simulink model "SimpleEKF_2007a"  (Simulink 6.6)
settings: Solver=FixedStepDiscrete  StartTime=0.0  StopTime=300  FixedStep=0.01  RelTol=1e-3
values from neighbouring files (symbols this model uses):
  initP = diag([ 1 1 1 1e5 1e5 1 1e5 1e5 1e5 ])    [SimpleEKF_init.m.m]
undefined symbols (not defined in the file or in its folder): DiscIntNeverNeededParam, gcbh, hwbcalib_subsystem
libraries: simulink x8, dspmtrx3 x5, dspinverses x1
(part 9 of 9)

== system SimpleEKF_2007a/INS/Attitude update/Stage2/Subsystem/a21/product1 ==
  1 : Inport  OutDataType=fixdt(1,16,0)  OutScaling=[]
  2 : Inport  Port=2  OutDataType=fixdt(1,16,0)  OutScaling=[]
  Product_1 : Product  OutDataType=fixdt(1,16,0)  OutScaling=[]  RndMeth=Zero  InputSameDT=on
  1000 : Outport  OutDataType=fixdt(1,16,0)  OutScaling=[]
  wires:
  Product_1/1 -> 1000/1
  1/1 -> Product_1/1
  2/1 -> Product_1/2

== system SimpleEKF_2007a/INS/Attitude update/Stage2/Subsystem/a21/sum ==
  1 : Inport  OutDataType=fixdt(1,16,0)  OutScaling=[]
  2 : Inport  Port=2  OutDataType=fixdt(1,16,0)  OutScaling=[]
  Sum_1 : Sum  Inputs=-+  OutDataType=fixdt(1,16,0)  OutScaling=[]  RndMeth=Zero  InputSameDT=on
  1000 : Outport  OutDataType=fixdt(1,16,0)  OutScaling=[]
  wires:
  Sum_1/1 -> 1000/1
  1/1 -> Sum_1/1
  2/1 -> Sum_1/2

== system SimpleEKF_2007a/INS/Attitude update/Stage2/Subsystem/a22/BorderBottom ==

== system SimpleEKF_2007a/INS/Attitude update/Stage2/Subsystem/a22/BorderLeft ==

== system SimpleEKF_2007a/INS/Attitude update/Stage2/Subsystem/a22/BorderRight ==

== system SimpleEKF_2007a/INS/Attitude update/Stage2/Subsystem/a22/BorderTop ==

== system SimpleEKF_2007a/INS/Attitude update/Stage2/Subsystem/a22/Subsystem Revision ==

== system SimpleEKF_2007a/INS/Attitude update/Stage2/Subsystem/a22/deMux ==
  Dmx : Inport  OutDataType=fixdt(1,16,0)  OutScaling=[]
  999 : Demux
  1 : Outport  OutDataType=fixdt(1,16,0)  OutScaling=[]
  2 : Outport  Port=2  OutDataType=fixdt(1,16,0)  OutScaling=[]
  3 : Outport  Port=3  OutDataType=fixdt(1,16,0)  OutScaling=[]
  4 : Outport  Port=4  OutDataType=fixdt(1,16,0)  OutScaling=[]
  wires:
  999/1 -> 1/1
  999/2 -> 2/1
  Dmx/1 -> 999/1
  999/3 -> 3/1
  999/4 -> 4/1

== system SimpleEKF_2007a/INS/Attitude update/Stage2/Subsystem/a22/product ==
  1 : Inport  OutDataType=fixdt(1,16,0)  OutScaling=[]
  2 : Inport  Port=2  OutDataType=fixdt(1,16,0)  OutScaling=[]
  Product_1 : Product  OutDataType=fixdt(1,16,0)  OutScaling=[]  RndMeth=Zero  InputSameDT=on
  1000 : Outport  OutDataType=fixdt(1,16,0)  OutScaling=[]
  wires:
  Product_1/1 -> 1000/1
  1/1 -> Product_1/1
  2/1 -> Product_1/2

== system SimpleEKF_2007a/INS/Attitude update/Stage2/Subsystem/a22/product1 ==
  1 : Inport  OutDataType=fixdt(1,16,0)  OutScaling=[]
  2 : Inport  Port=2  OutDataType=fixdt(1,16,0)  OutScaling=[]
  Product_1 : Product  OutDataType=fixdt(1,16,0)  OutScaling=[]  RndMeth=Zero  InputSameDT=on
  1000 : Outport  OutDataType=fixdt(1,16,0)  OutScaling=[]
  wires:
  Product_1/1 -> 1000/1
  1/1 -> Product_1/1
  2/1 -> Product_1/2

== system SimpleEKF_2007a/INS/Attitude update/Stage2/Subsystem/a22/product2 ==
  1 : Inport  OutDataType=fixdt(1,16,0)  OutScaling=[]
  2 : Inport  Port=2  OutDataType=fixdt(1,16,0)  OutScaling=[]
  Product_1 : Product  OutDataType=fixdt(1,16,0)  OutScaling=[]  RndMeth=Zero  InputSameDT=on
  1000 : Outport  OutDataType=fixdt(1,16,0)  OutScaling=[]
  wires:
  Product_1/1 -> 1000/1
  1/1 -> Product_1/1
  2/1 -> Product_1/2

== system SimpleEKF_2007a/INS/Attitude update/Stage2/Subsystem/a22/product3 ==
  1 : Inport  OutDataType=fixdt(1,16,0)  OutScaling=[]
  2 : Inport  Port=2  OutDataType=fixdt(1,16,0)  OutScaling=[]
  Product_1 : Product  OutDataType=fixdt(1,16,0)  OutScaling=[]  RndMeth=Zero  InputSameDT=on
  1000 : Outport  OutDataType=fixdt(1,16,0)  OutScaling=[]
  wires:
  Product_1/1 -> 1000/1
  1/1 -> Product_1/1
  2/1 -> Product_1/2

== system SimpleEKF_2007a/INS/Attitude update/Stage2/Subsystem/a22/sum ==
  1 : Inport  OutDataType=fixdt(1,16,0)  OutScaling=[]
  2 : Inport  Port=2  OutDataType=fixdt(1,16,0)  OutScaling=[]
  3 : Inport  Port=3  OutDataType=fixdt(1,16,0)  OutScaling=[]
  4 : Inport  Port=4  OutDataType=fixdt(1,16,0)  OutScaling=[]
  Sum_1 : Sum  Inputs=+-+-  OutDataType=fixdt(1,16,0)  OutScaling=[]  RndMeth=Zero  InputSameDT=on
  1000 : Outport  OutDataType=fixdt(1,16,0)  OutScaling=[]
  wires:
  Sum_1/1 -> 1000/1
  1/1 -> Sum_1/1
  2/1 -> Sum_1/2
  3/1 -> Sum_1/3
  4/1 -> Sum_1/4

== system SimpleEKF_2007a/INS/Attitude update/Stage2/Subsystem/a23/BorderBottom ==

== system SimpleEKF_2007a/INS/Attitude update/Stage2/Subsystem/a23/BorderLeft ==

== system SimpleEKF_2007a/INS/Attitude update/Stage2/Subsystem/a23/BorderRight ==

== system SimpleEKF_2007a/INS/Attitude update/Stage2/Subsystem/a23/BorderTop ==

== system SimpleEKF_2007a/INS/Attitude update/Stage2/Subsystem/a23/Subsystem Revision ==

== system SimpleEKF_2007a/INS/Attitude update/Stage2/Subsystem/a23/deMux ==
  Dmx : Inport  OutDataType=fixdt(1,16,0)  OutScaling=[]
  999 : Demux
  1 : Outport  OutDataType=fixdt(1,16,0)  OutScaling=[]
  2 : Outport  Port=2  OutDataType=fixdt(1,16,0)  OutScaling=[]
  3 : Outport  Port=3  OutDataType=fixdt(1,16,0)  OutScaling=[]
  4 : Outport  Port=4  OutDataType=fixdt(1,16,0)  OutScaling=[]
  wires:
  999/1 -> 1/1
  999/2 -> 2/1
  Dmx/1 -> 999/1
  999/3 -> 3/1
  999/4 -> 4/1

== system SimpleEKF_2007a/INS/Attitude update/Stage2/Subsystem/a23/gain ==
  1 : Inport  OutDataType=fixdt(1,16,0)  OutScaling=[]
  Gain_1 : Gain  Gain=eval(gain)  ParameterDataType=fixdt(1,16,0)  ParameterScaling=[]  OutDataType=fixdt(1,16,0)  OutScaling=[]  RndMeth=Zero
  2 : Outport  OutDataType=fixdt(1,16,0)  OutScaling=[]
  wires:
  1/1 -> Gain_1/1
  Gain_1/1 -> 2/1

== system SimpleEKF_2007a/INS/Attitude update/Stage2/Subsystem/a23/product ==
  1 : Inport  OutDataType=fixdt(1,16,0)  OutScaling=[]
  2 : Inport  Port=2  OutDataType=fixdt(1,16,0)  OutScaling=[]
  Product_1 : Product  OutDataType=fixdt(1,16,0)  OutScaling=[]  RndMeth=Zero  InputSameDT=on
  1000 : Outport  OutDataType=fixdt(1,16,0)  OutScaling=[]
  wires:
  Product_1/1 -> 1000/1
  1/1 -> Product_1/1
  2/1 -> Product_1/2

== system SimpleEKF_2007a/INS/Attitude update/Stage2/Subsystem/a23/product1 ==
  1 : Inport  OutDataType=fixdt(1,16,0)  OutScaling=[]
  2 : Inport  Port=2  OutDataType=fixdt(1,16,0)  OutScaling=[]
  Product_1 : Product  OutDataType=fixdt(1,16,0)  OutScaling=[]  RndMeth=Zero  InputSameDT=on
  1000 : Outport  OutDataType=fixdt(1,16,0)  OutScaling=[]
  wires:
  Product_1/1 -> 1000/1
  1/1 -> Product_1/1
  2/1 -> Product_1/2

== system SimpleEKF_2007a/INS/Attitude update/Stage2/Subsystem/a23/sum ==
  1 : Inport  OutDataType=fixdt(1,16,0)  OutScaling=[]
  2 : Inport  Port=2  OutDataType=fixdt(1,16,0)  OutScaling=[]
  Sum_1 : Sum  OutDataType=fixdt(1,16,0)  OutScaling=[]  RndMeth=Zero  InputSameDT=on
  1000 : Outport  OutDataType=fixdt(1,16,0)  OutScaling=[]
  wires:
  Sum_1/1 -> 1000/1
  1/1 -> Sum_1/1
  2/1 -> Sum_1/2

== system SimpleEKF_2007a/INS/Attitude update/Stage2/Subsystem/a31/BorderBottom ==

== system SimpleEKF_2007a/INS/Attitude update/Stage2/Subsystem/a31/BorderLeft ==

== system SimpleEKF_2007a/INS/Attitude update/Stage2/Subsystem/a31/BorderRight ==

== system SimpleEKF_2007a/INS/Attitude update/Stage2/Subsystem/a31/BorderTop ==

== system SimpleEKF_2007a/INS/Attitude update/Stage2/Subsystem/a31/Subsystem Revision ==

== system SimpleEKF_2007a/INS/Attitude update/Stage2/Subsystem/a31/deMux ==
  Dmx : Inport  OutDataType=fixdt(1,16,0)  OutScaling=[]
  999 : Demux
  1 : Outport  OutDataType=fixdt(1,16,0)  OutScaling=[]
  2 : Outport  Port=2  OutDataType=fixdt(1,16,0)  OutScaling=[]
  3 : Outport  Port=3  OutDataType=fixdt(1,16,0)  OutScaling=[]
  4 : Outport  Port=4  OutDataType=fixdt(1,16,0)  OutScaling=[]
  wires:
  999/1 -> 1/1
  999/2 -> 2/1
  Dmx/1 -> 999/1
  999/3 -> 3/1
  999/4 -> 4/1

== system SimpleEKF_2007a/INS/Attitude update/Stage2/Subsystem/a31/gain ==
  1 : Inport  OutDataType=fixdt(1,16,0)  OutScaling=[]
  Gain_1 : Gain  Gain=eval(gain)  ParameterDataType=fixdt(1,16,0)  ParameterScaling=[]  OutDataType=fixdt(1,16,0)  OutScaling=[]  RndMeth=Zero
  2 : Outport  OutDataType=fixdt(1,16,0)  OutScaling=[]
  wires:
  1/1 -> Gain_1/1
  Gain_1/1 -> 2/1

== system SimpleEKF_2007a/INS/Attitude update/Stage2/Subsystem/a31/product ==
  1 : Inport  OutDataType=fixdt(1,16,0)  OutScaling=[]
  2 : Inport  Port=2  OutDataType=fixdt(1,16,0)  OutScaling=[]
  Product_1 : Product  OutDataType=fixdt(1,16,0)  OutScaling=[]  RndMeth=Zero  InputSameDT=on
  1000 : Outport  OutDataType=fixdt(1,16,0)  OutScaling=[]
  wires:
  Product_1/1 -> 1000/1
  1/1 -> Product_1/1
  2/1 -> Product_1/2

== system SimpleEKF_2007a/INS/Attitude update/Stage2/Subsystem/a31/product1 ==
  1 : Inport  OutDataType=fixdt(1,16,0)  OutScaling=[]
  2 : Inport  Port=2  OutDataType=fixdt(1,16,0)  OutScaling=[]
  Product_1 : Product  OutDataType=fixdt(1,16,0)  OutScaling=[]  RndMeth=Zero  InputSameDT=on
  1000 : Outport  OutDataType=fixdt(1,16,0)  OutScaling=[]
  wires:
  Product_1/1 -> 1000/1
  1/1 -> Product_1/1
  2/1 -> Product_1/2

== system SimpleEKF_2007a/INS/Attitude update/Stage2/Subsystem/a31/sum ==
  1 : Inport  OutDataType=fixdt(1,16,0)  OutScaling=[]
  2 : Inport  Port=2  OutDataType=fixdt(1,16,0)  OutScaling=[]
  Sum_1 : Sum  OutDataType=fixdt(1,16,0)  OutScaling=[]  RndMeth=Zero  InputSameDT=on
  1000 : Outport  OutDataType=fixdt(1,16,0)  OutScaling=[]
  wires:
  Sum_1/1 -> 1000/1
  1/1 -> Sum_1/1
  2/1 -> Sum_1/2

== system SimpleEKF_2007a/INS/Attitude update/Stage2/Subsystem/a32/BorderBottom ==

== system SimpleEKF_2007a/INS/Attitude update/Stage2/Subsystem/a32/BorderLeft ==

== system SimpleEKF_2007a/INS/Attitude update/Stage2/Subsystem/a32/BorderRight ==

== system SimpleEKF_2007a/INS/Attitude update/Stage2/Subsystem/a32/BorderTop ==

== system SimpleEKF_2007a/INS/Attitude update/Stage2/Subsystem/a32/Subsystem Revision ==

== system SimpleEKF_2007a/INS/Attitude update/Stage2/Subsystem/a32/deMux ==
  Dmx : Inport  OutDataType=fixdt(1,16,0)  OutScaling=[]
  999 : Demux
  1 : Outport  OutDataType=fixdt(1,16,0)  OutScaling=[]
  2 : Outport  Port=2  OutDataType=fixdt(1,16,0)  OutScaling=[]
  3 : Outport  Port=3  OutDataType=fixdt(1,16,0)  OutScaling=[]
  4 : Outport  Port=4  OutDataType=fixdt(1,16,0)  OutScaling=[]
  wires:
  999/1 -> 1/1
  999/2 -> 2/1
  Dmx/1 -> 999/1
  999/3 -> 3/1
  999/4 -> 4/1

== system SimpleEKF_2007a/INS/Attitude update/Stage2/Subsystem/a32/gain ==
  1 : Inport  OutDataType=fixdt(1,16,0)  OutScaling=[]
  Gain_1 : Gain  Gain=eval(gain)  ParameterDataType=fixdt(1,16,0)  ParameterScaling=[]  OutDataType=fixdt(1,16,0)  OutScaling=[]  RndMeth=Zero
  2 : Outport  OutDataType=fixdt(1,16,0)  OutScaling=[]
  wires:
  1/1 -> Gain_1/1
  Gain_1/1 -> 2/1

== system SimpleEKF_2007a/INS/Attitude update/Stage2/Subsystem/a32/product ==
  1 : Inport  OutDataType=fixdt(1,16,0)  OutScaling=[]
  2 : Inport  Port=2  OutDataType=fixdt(1,16,0)  OutScaling=[]
  Product_1 : Product  OutDataType=fixdt(1,16,0)  OutScaling=[]  RndMeth=Zero  InputSameDT=on
  1000 : Outport  OutDataType=fixdt(1,16,0)  OutScaling=[]
  wires:
  Product_1/1 -> 1000/1
  1/1 -> Product_1/1
  2/1 -> Product_1/2

== system SimpleEKF_2007a/INS/Attitude update/Stage2/Subsystem/a32/product1 ==
  1 : Inport  OutDataType=fixdt(1,16,0)  OutScaling=[]
  2 : Inport  Port=2  OutDataType=fixdt(1,16,0)  OutScaling=[]
  Product_1 : Product  OutDataType=fixdt(1,16,0)  OutScaling=[]  RndMeth=Zero  InputSameDT=on
  1000 : Outport  OutDataType=fixdt(1,16,0)  OutScaling=[]
  wires:
  Product_1/1 -> 1000/1
  1/1 -> Product_1/1
  2/1 -> Product_1/2

== system SimpleEKF_2007a/INS/Attitude update/Stage2/Subsystem/a32/sum ==
  1 : Inport  OutDataType=fixdt(1,16,0)  OutScaling=[]
  2 : Inport  Port=2  OutDataType=fixdt(1,16,0)  OutScaling=[]
  Sum_1 : Sum  Inputs=-+  OutDataType=fixdt(1,16,0)  OutScaling=[]  RndMeth=Zero  InputSameDT=on
  1000 : Outport  OutDataType=fixdt(1,16,0)  OutScaling=[]
  wires:
  Sum_1/1 -> 1000/1
  1/1 -> Sum_1/1
  2/1 -> Sum_1/2

== system SimpleEKF_2007a/INS/Attitude update/Stage2/Subsystem/a33/BorderBottom ==

== system SimpleEKF_2007a/INS/Attitude update/Stage2/Subsystem/a33/BorderLeft ==

== system SimpleEKF_2007a/INS/Attitude update/Stage2/Subsystem/a33/BorderRight ==

== system SimpleEKF_2007a/INS/Attitude update/Stage2/Subsystem/a33/BorderTop ==

== system SimpleEKF_2007a/INS/Attitude update/Stage2/Subsystem/a33/Subsystem Revision ==

== system SimpleEKF_2007a/INS/Attitude update/Stage2/Subsystem/a33/deMux ==
  Dmx : Inport  OutDataType=fixdt(1,16,0)  OutScaling=[]
  999 : Demux
  1 : Outport  OutDataType=fixdt(1,16,0)  OutScaling=[]
  2 : Outport  Port=2  OutDataType=fixdt(1,16,0)  OutScaling=[]
  3 : Outport  Port=3  OutDataType=fixdt(1,16,0)  OutScaling=[]
  4 : Outport  Port=4  OutDataType=fixdt(1,16,0)  OutScaling=[]
  wires:
  999/1 -> 1/1
  999/2 -> 2/1
  Dmx/1 -> 999/1
  999/3 -> 3/1
  999/4 -> 4/1

== system SimpleEKF_2007a/INS/Attitude update/Stage2/Subsystem/a33/product ==
  1 : Inport  OutDataType=fixdt(1,16,0)  OutScaling=[]
  2 : Inport  Port=2  OutDataType=fixdt(1,16,0)  OutScaling=[]
  Product_1 : Product  OutDataType=fixdt(1,16,0)  OutScaling=[]  RndMeth=Zero  InputSameDT=on
  1000 : Outport  OutDataType=fixdt(1,16,0)  OutScaling=[]
  wires:
  Product_1/1 -> 1000/1
  1/1 -> Product_1/1
  2/1 -> Product_1/2

== system SimpleEKF_2007a/INS/Attitude update/Stage2/Subsystem/a33/product1 ==
  1 : Inport  OutDataType=fixdt(1,16,0)  OutScaling=[]
  2 : Inport  Port=2  OutDataType=fixdt(1,16,0)  OutScaling=[]
  Product_1 : Product  OutDataType=fixdt(1,16,0)  OutScaling=[]  RndMeth=Zero  InputSameDT=on
  1000 : Outport  OutDataType=fixdt(1,16,0)  OutScaling=[]
  wires:
  Product_1/1 -> 1000/1
  1/1 -> Product_1/1
  2/1 -> Product_1/2

== system SimpleEKF_2007a/INS/Attitude update/Stage2/Subsystem/a33/product2 ==
  1 : Inport  OutDataType=fixdt(1,16,0)  OutScaling=[]
  2 : Inport  Port=2  OutDataType=fixdt(1,16,0)  OutScaling=[]
  Product_1 : Product  OutDataType=fixdt(1,16,0)  OutScaling=[]  RndMeth=Zero  InputSameDT=on
  1000 : Outport  OutDataType=fixdt(1,16,0)  OutScaling=[]
  wires:
  Product_1/1 -> 1000/1
  1/1 -> Product_1/1
  2/1 -> Product_1/2

== system SimpleEKF_2007a/INS/Attitude update/Stage2/Subsystem/a33/product3 ==
  1 : Inport  OutDataType=fixdt(1,16,0)  OutScaling=[]
  2 : Inport  Port=2  OutDataType=fixdt(1,16,0)  OutScaling=[]
  Product_1 : Product  OutDataType=fixdt(1,16,0)  OutScaling=[]  RndMeth=Zero  InputSameDT=on
  1000 : Outport  OutDataType=fixdt(1,16,0)  OutScaling=[]
  wires:
  Product_1/1 -> 1000/1
  1/1 -> Product_1/1
  2/1 -> Product_1/2

== system SimpleEKF_2007a/INS/Attitude update/Stage2/Subsystem/a33/sum ==
  1 : Inport  OutDataType=fixdt(1,16,0)  OutScaling=[]
  2 : Inport  Port=2  OutDataType=fixdt(1,16,0)  OutScaling=[]
  3 : Inport  Port=3  OutDataType=fixdt(1,16,0)  OutScaling=[]
  4 : Inport  Port=4  OutDataType=fixdt(1,16,0)  OutScaling=[]
  Sum_1 : Sum  Inputs=+--+  OutDataType=fixdt(1,16,0)  OutScaling=[]  RndMeth=Zero  InputSameDT=on
  1000 : Outport  OutDataType=fixdt(1,16,0)  OutScaling=[]
  wires:
  Sum_1/1 -> 1000/1
  1/1 -> Sum_1/1
  2/1 -> Sum_1/2
  3/1 -> Sum_1/3
  4/1 -> Sum_1/4

== system SimpleEKF_2007a/INS/Attitude update/Stage2/Subsystem/quat normalize/qat modulus ==
  q : Inport  OutDataType=fixdt(1,16,0)  OutScaling=[]
  Demux : Demux
  Math Function : Math  Operator=sqrt  OutDataType=fixdt(1,16,0)  OutScaling=[]  SaturateOnIntegerOverflow=on
  Product{,1..3} (4 alike) : Product  OutDataType=fixdt(1,16,0)  OutScaling=[]
  Sum : Sum  Inputs=4  OutDataType=fixdt(1,16,0)  OutScaling=[]
  |q| : Outport  OutDataType=fixdt(1,16,0)  OutScaling=[]
  wires:
  Math Function/1 -> |q|/1
  Demux/4 -> Product3/1, Product3/2
  Demux/3 -> Product2/1, Product2/2
  Demux/2 -> Product1/1, Product1/2
  Demux/1 -> Product/1, Product/2
  Product3/1 -> Sum/4
  Product2/1 -> Sum/3
  Product1/1 -> Sum/2
  Product/1 -> Sum/1
  Sum/1 -> Math Function/1
  q/1 -> Demux/1

== matlab function EKF/MeasureVector/MATLAB Function ==
  data: posIns input double; posGps input double; y output double; velIns input double; velGps input double
function y = fcn(posIns,posGps,velIns,velGps)

y=[posIns-posGps;velIns-velGps];

== matlab function EKF/MATLAB Function ==
  data: g0 input double; wNavToEciInNav input double; posLat input double; h input double; dcmBodyToNav input double; velNorth input double; velEast input double; velDown input double; y input double; accNav input double; x_prev input double; P_prev input double; x output double; P output double
function [x,P] = EKF(g0,wNavToEciInNav,posLat,h,dcmBodyToNav,velNorth,velEast,velDown,y,accNav,x_prev,P_prev)
%omega=wNavToEciInNav
%f21 x,y,z- demuxed prouct of dcmBodyToNav and accelerometer output
%g0 third item of gravity vector. eq. 2.85
%rGeo - geocentrric radius of the surface, eq.2.88
%RN meridian radius of curvature, eq. 2.65
%RE transverse radius of curvature, eq. 2.66
R0=6378137;
e=0.0818191908425;
RN=R0*(1-e^2)/((1-(e^2*sin(posLat)))^1.5);
RE=R0/sqrt(1-(e^2*sin(posLat)));
rGeo=RE*sqrt(cos(posLat)^2+((1-e^2)^2*sin(posLat)^2));
omegaie=7.2921158e-5;

O=[0 0 0;
   0 0 0;
   0 0 0];
Fc11=-wNavToEciInNav;
Fc1211=0;
Fc1212=(-1/(RE+h));
Fc1213=0;
Fc1221=(1/(RN+h));
Fc1222=0;
Fc1223=0;
Fc1231=0;
Fc1232=(((tan(posLat))/(RE+h)));
Fc1233=0;
Fc12=[Fc1211 Fc1212 Fc1213;Fc1221 Fc1222 Fc1223;Fc1231 Fc1232 Fc1233];

Fc1311=omegaie*sin(posLat);
Fc1312=0;
Fc1313=((velEast/(RE+h)^2));
Fc1321=0;
Fc1322=0;
Fc1323=((-velNorth/(RN+h)^2));
Fc1331=omegaie*cos(posLat)+((velEast/((RE+h)*cos(posLat)^2)));
Fc1332=0;
Fc1333=((-velEast*tan(posLat)/(RE+h)^2));
Fc13=[Fc1311 Fc1312 Fc1313;Fc1321 Fc1322 Fc1323;Fc1331 Fc1332 Fc1333];




  Fc2311a=-((velEast)^2)/((RE+h)*cos(posLat)^2);
         Fc2311b=-2*velEast*omegaie*cos(posLat);
    Fc2311=Fc2311a+Fc2311b;
    Fc2312=0;
         Fc2313a=((velEast^2)*tan(posLat))/((RE+h)^2);
         Fc2313b=-(velNorth*velDown)/((RN+h)^2);
    Fc2313=Fc2313a+Fc2313b;
         Fc2321a=(velEast*velNorth)/((RE+h)*(cos(posLat)^2));
         Fc2321b=2*velNorth*omegaie*cos(posLat);
         Fc2321c=-2*velDown*omegaie*sin(posLat);
    Fc2321=Fc2321a+Fc2321b+Fc2321c;
    
    Fc2322=0;
    Fc2323a=(-velNorth*velEast*tan(posLat))-((velEast*velDown));
    Fc2323=Fc2323a/((RE+h)^2);
    Fc2331=2*velEast*omegaie*sin(posLat);
    Fc2332=0;
    Fc2333=(velEast^2/((RE+h)^2)+((velNorth^2)/((RN+h)^2))-(2*g0/rGeo));
Fc23=[Fc2311 Fc2312 Fc2313;Fc2321 Fc2322 Fc2323;Fc2331 Fc2332 Fc2333];


    Fc2211=(velDown/(RN+h));
    Fc2212=(((-2*velEast*tan(posLat))/(RE+h))-2*omegaie*sin(posLat));
    Fc2213=(velNorth/(RN+h));
    Fc2221=(((velEast*tan(posLat))/(RE+h))+2*omegaie*sin(posLat));
    Fc2222=((velNorth*tan(posLat)+velDown)/(RE+h));
    Fc2223=(velEast/(RE+h)+(2*omegaie*cos(posLat)));
    Fc2231=(-2*velNorth/(RN+h));
    Fc2232=(((-2*velEast)/(RE+h))-(2*omegaie*cos(posLat)));
    Fc2233=0;
   Fc22=[Fc2211 Fc2212 Fc2213;Fc2221 Fc2222 Fc2223;Fc2231 Fc2232 Fc2233];
    

Fc21=-accNav;                         %acc.output in NAV frame

Fc3211=1/(RN+h);
Fc3212=0;
Fc3213=0;
Fc3221=0;
Fc3222=1/((RE+h)*cos(posLat));
Fc3223=0;
Fc3231=0;
Fc3232=0;
Fc3233=-1;
Fc32=[Fc3211 Fc3212 Fc3213;Fc3221 Fc3222 Fc3223;Fc3231 Fc3232 Fc3233];

Fc3313=-velNorth/((RN+h)^2);
Fc3321=(velEast*sin(posLat))/((RE+h)*cos(posLat)^2);
Fc3323=velEast/((RE+h)^2*cos(posLat));
Fc33=[0 0 Fc3313;Fc3321 0 Fc3323; 0 0 0];


Fc=[Fc22 Fc23 dcmBodyToNav;
    Fc32 Fc33 O;
    O O O];
dt = 0.01;

F = eye(9)+Fc*dt+(Fc*dt).^2/factorial(2)+(Fc*dt).^3/factorial(3);

accVarX=0.00003;
accVarY=0.00003;
accVarZ=0.00003;
gyrVarX=0;
gyrVarY=0;
gyrVarZ=0;

Qc =[accVarX 0 0 ;
    0 accVarY 0 ;
    0 0 accVarZ ];

G=[dcmBodyToNav(1,1) dcmBodyToNav(1,2) dcmBodyToNav(1,3) ;
   dcmBodyToNav(2,1) dcmBodyToNav(2,2) dcmBodyToNav(2,3) ;
   dcmBodyToNav(3,1) dcmBodyToNav(3,2) dcmBodyToNav(3,3) ;
   0 0 0 ;
   0 0 0 ;
   0 0 0 ;
   0 0 0 ;
   0 0 0 ;
   0 0 0 ];
   
     
Q = 0.5*(F*G*Qc*G'+G*Qc*G'*F')*dt;

R = [1e-12 0 0 0 0 0;
    0 1e-12 0 0 0 0;
    0 0 2.5 0 0 0;
    0 0 0 0.0001 0 0;
    0 0 0 0 0.0001 0;
    0 0 0 0 0 0.0001];  

H = [0 0 0 0 1 0 0 0 0 ;
     0 0 0 1 0 0 0 0 0 ;
     0 0 0 0 0 1 0 0 0 ;
     1 0 0 0 0 0 0 0 0 ;
     0 1 0 0 0 0 0 0 0 ;
     0 0 1 0 0 0 0 0 0 ];
% -----------------------------------------------------------
x_prev = [0;0;0;0;0;0;0;0;0];

x_hat = F*x_prev;
P_hat = F*P_prev*F'+Q;
K = (P_hat*H')/(H*P_hat*H'+R);

x = x_hat+K*(y-H*x_hat);
P = (eye(9)-K*H)*P_hat*(eye(9)-K*H)'+K*R*K';

== matlab function Display results/MATLAB Function ==
  data: lambda output double; l input inherited
function lambda = myWrapToPi(l)
    if (pi < l )
         a=pi-l;
         lambda=l-2*pi;
    else
        lambda=l;
end
